simulink model "task2a_j"  (R2019a)
settings: Solver=VariableStepAuto  StartTime=0  StopTime=10  RelTol=1e-3
settings Model: Creator=Artem  LastModifiedBy=Artem

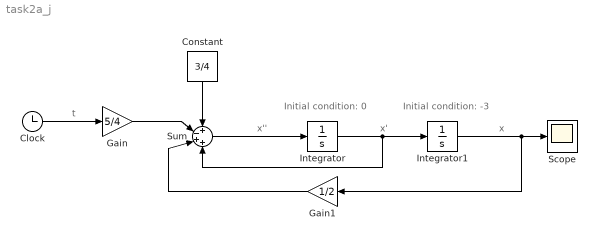
== system task2a_j ==
  note: x''
  note: t
  note: Initial condition: -3
  note: Initial condition: 0
  note: x
  note: x'
  Clock : Clock
  Constant : Constant  Value=3/4
  Gain : Gain  Gain=5/4
  Gain1 : Gain  Gain=1/2
  Integrator : Integrator
  Integrator1 : Integrator  InitialCondition=-3
  Scope : Scope
  Sum : Sum  Inputs=+-++
  wires:
  Integrator1/1 -> Gain1/1, Scope/1
  Sum/1 -> Integrator/1
  Constant/1 -> Sum/1
  Integrator/1 -> Integrator1/1, Sum/4
  Gain1/1 -> Sum/3
  Clock/1 -> Gain/1
  Gain/1 -> Sum/2
